simulink model "Cp_Lambda_Calculation"  (R2025a)
settings: Solver=FixedStepDiscrete  StartTime=0.0  StopTime=0  RelTol=1e-3
settings Model: Creator=Venkatesh  LastModifiedBy=lcrsb
settings SolverCC: AlgebraicLoopSolver=TrustRegion
settings DataIOCC: LimitDataPoints=on  SaveFormat=Array  ReturnWorkspaceOutputs=off
settings OptimizationCC: DefaultParameterBehavior=Inlined  UseDivisionForNetSlopeComputation=on  GainParamInheritBuiltInType=on  UseFloatMulNetSlope=on  InlineInvariantSignals=on  PassReuseOutputArgsAs=Individual arguments  ZeroExternalMemoryAtStartup=off  ZeroInternalMemoryAtStartup=off  NoFixptDivByZeroProtection=on  EfficientFloat2IntCast=on  LifeSpan=1  OptimizeBlockOrder=speed  DifferentSizesBufferReuse=on  EfficientTunableParamExpr=on
settings DebuggingCC: ParameterTunabilityLossMsg=error  UnconnectedInputMsg=warning  UnconnectedOutputMsg=warning  UnconnectedLineMsg=warning  SFUnexpectedBacktrackingDiag=warning  SFNoUnconditionalDefaultTransitionDiag=warning  SFExecutionAtInitializationDiag=none  ArithmeticOperatorsInVariantConditions=warning
settings HardwareCC: ProdLongLongMode=on
settings ModelReferenceCC: PropagateSignalLabelsOutOfModel=off
settings SFSimCC: SimUseLocalCustomCode=off  MATLABDynamicMemAlloc=off  CustomCodeUndefinedFunction=UseInterfaceOnly
settings RTWCC: SystemTargetFile=ert.tlc  TemplateMakefile=ert_default_tmf  RTWUseLocalCustomCode=off  GPUComputeCapability=3.5  Description=Embedded Coder
settings CodeAppCC: ForceParamTrailComments=on  IgnoreCustomStorageClasses=off  OperatorAnnotations=on  SimulinkDataObjDesc=on  SFDataObjDesc=on  CustomSymbolStrGlobalVar=rt$N$M  CustomSymbolStrType=$N$M  CustomSymbolStrFcn=$N$M$F  CustomSymbolStrMacro=$N$M  InsertBlockDesc=on
settings ERTTargetCC: ExtModeTransport=0.0  ExtModeStaticAlloc=off  ExtModeMexFile=ext_comm  ExtModeIntrfLevel=Level1  ERTCustomFileTemplate=example_file_process.tlc  ERTFilePackagingFormat=CompactWithDataFile  GenerateSampleERTMain=on  IncludeMdlTerminateFcn=off  CombineSignalStateStructs=on  SuppressErrorStatus=on  SupportAbsoluteTime=off  SupportComplex=off
settings ConfigComp: CovMetricSettings=dw  CovSaveCumulativeToWorkspaceVar=on  CovSaveSingleToWorkspaceVar=on  CovExternalEMLEnable=off  CovSFcnEnable=off

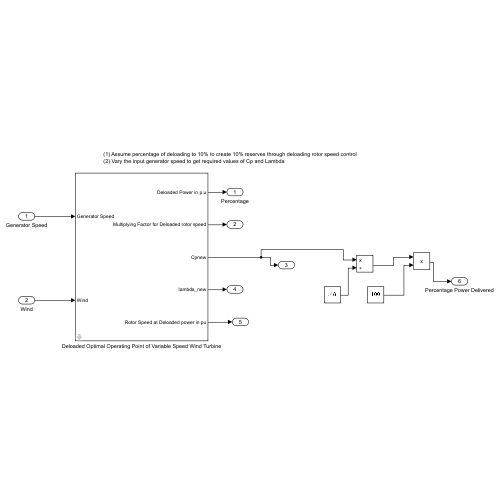
[thumbnail: Simulink's stored preview of the top-level diagram]
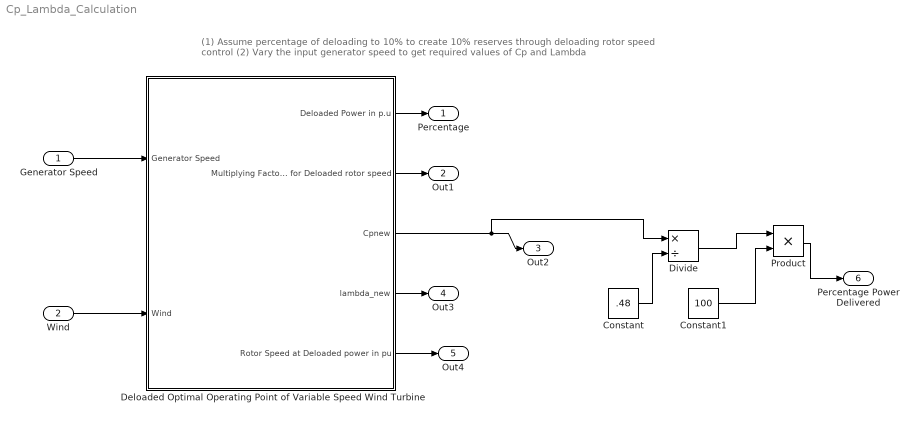
== system Cp_Lambda_Calculation ==
  note: (1) Assume percentage of deloading to 10% to create 10% reserves through deloading rotor speed control
      | (2) Vary the input generator speed to get required values of Cp and Lambda
  Generator Speed : Inport
  Wind : Inport  Port=2
  Constant : Constant  Value=.48
  Constant1 : Constant  Value=100
  Deloaded Optimal Operating Point of Variable Speed Wind Turbine : Subsystem  mask(Deloaded Optimal Operating Point Calculation){per_del=10, Generator_Speed=1.4207, Wind_Speed=12, Speed_MPPT=1.2, cp_opt=.4781, lambda_opt=8.3869, wind_base=12, speed_nom=1.2, lambda_nom=8.1, cp_nom=.48, beta=0}
      mask prompts: per_del "Percentage of Deloading"; Generator_Speed "Measured/Input Generator Speed p.u."; Wind_Speed "Wind Speed in m/s"; Speed_MPPT "Rotor Speed at MPPT in pu"; cp_opt "Optimum Power Coefficient"; lambda_opt "Optimum Tip Speed Ratio"; wind_base "Base Wind Speed in m/s"; speed_nom "Nominal Generator Speed p.u."; lambda_nom "Nominal Tip Speed Ratio"; cp_nom "Nominal Power Coefficient"; beta "Pitch Angle in degrees"
      mask help:
      | This block calculates the inputs required for the equation# 23 taken from the following reference:
      | []R.G. de Almeida, E. D. Castronuovo, and J. A. Peyas Lopes, “Optimum generation control in wind parks when carrying out system operator requests,” IEEE Trans. Power Syst., vol. 21, no. 2, pp. 718-725, May. 2006
  Divide : Product  Inputs=*/
  Product : Product
  Percentage : Outport
  Out1 : Outport  Port=2
  Out2 : Outport  Port=3
  Out3 : Outport  Port=4
  Out4 : Outport  Port=5
  Percentage Power Delivered : Outport  Port=6
  wires:
  Deloaded Optimal Operating Point of Variable Speed Wind Turbine/1(Deloaded Power in p.u) -> Percentage/1
  Deloaded Optimal Operating Point of Variable Speed Wind Turbine/2(Multiplying Factor for Deloaded rotor speed) -> Out1/1
  Deloaded Optimal Operating Point of Variable Speed Wind Turbine/3(Cpnew) -> Out2/1, Divide/1
  Deloaded Optimal Operating Point of Variable Speed Wind Turbine/4(lambda_new) -> Out3/1
  Deloaded Optimal Operating Point of Variable Speed Wind Turbine/5(Rotor Speed at Deloaded power in pu) -> Out4/1
  Constant/1 -> Divide/2
  Product/1 -> Percentage Power Delivered/1
  Divide/1 -> Product/1
  Constant1/1 -> Product/2
  Generator Speed/1 -> Deloaded Optimal Operating Point of Variable Speed Wind Turbine/1(Generator Speed)
  Wind/1 -> Deloaded Optimal Operating Point of Variable Speed Wind Turbine/2(Wind)

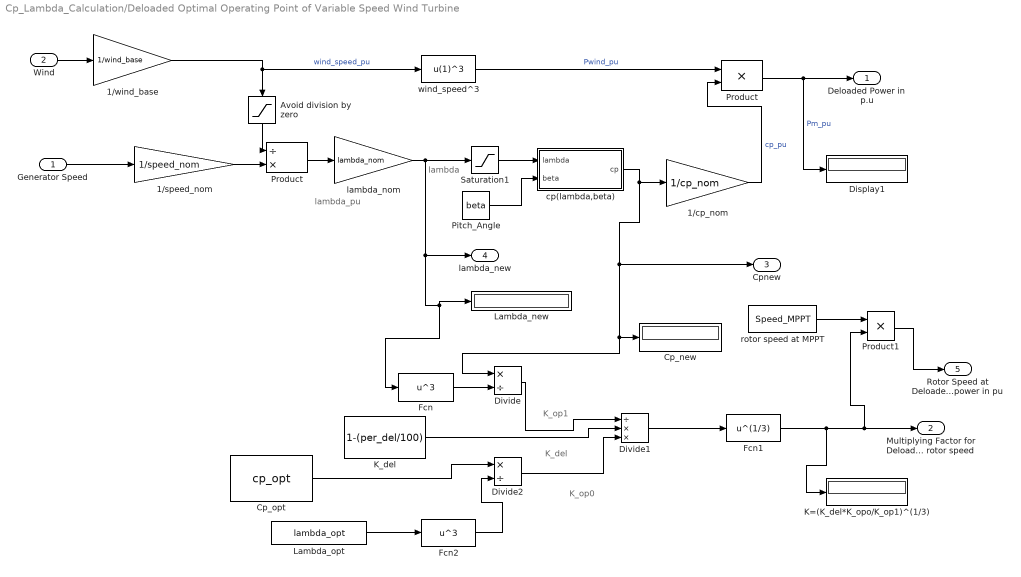
== system Cp_Lambda_Calculation/Deloaded Optimal Operating Point of Variable Speed Wind Turbine ==
  note: K_del
  note: K_op1
  note: K_op0
  note: lambda
  note: lambda_pu
  Generator Speed : Inport
  Wind : Inport  Port=2
  1/cp_nom : Gain  Gain=1/cp_nom  SaturateOnIntegerOverflow=on  OutDataTypeStr=Inherit: Same as input  ParamDataTypeStr=Inherit: Same as input
  "1/speed_nom " : Gain  Gain=1/speed_nom  SaturateOnIntegerOverflow=on  OutDataTypeStr=Inherit: Same as input  ParamDataTypeStr=Inherit: Same as input
  1/wind_base : Gain  Gain=1/wind_base  SaturateOnIntegerOverflow=on  OutDataTypeStr=Inherit: Same as input  ParamDataTypeStr=Inherit: Same as input
  "Avoid division by zero " : Saturate  UpperLimit=1e6  LowerLimit=1e-6
  Cp_new : Display
  Cp_opt : Constant  Value=cp_opt
  Display1 : Display
  Divide : Product  Inputs=*/
  Divide1 : Product  Inputs=/**
  Divide2 : Product  Inputs=*/
  Fcn : Fcn  Expr=u^3
  Fcn1 : Fcn  Expr=u^(1/3)
  Fcn2 : Fcn  Expr=u^3
  K=(K_del*K_opo/K_op1)^(1/3) : Display
  K_del : Constant  Value=1-(per_del/100)
  Lambda_new : Display
  Lambda_opt : Constant  Value=lambda_opt
  Pitch_Angle : Constant  Value=beta
  Product : Product  Inputs=/*  SaturateOnIntegerOverflow=on  OutDataTypeStr=Inherit: Same as first input
  "Product " : Product  SaturateOnIntegerOverflow=on  OutDataTypeStr=Inherit: Same as first input
  Product1 : Product
  Saturation1 : Saturate  UpperLimit=inf  LowerLimit=1e-6
  cp(lambda,beta) : Subsystem
  lambda_nom : Gain  Gain=lambda_nom  SaturateOnIntegerOverflow=on  OutDataTypeStr=Inherit: Same as input  ParamDataTypeStr=Inherit: Same as input
  rotor speed at MPPT : Constant  Value=Speed_MPPT
  wind_speed^3 : Fcn  Expr=u(1)^3
  Deloaded Power in p.u : Outport
  Multiplying Factor for Deloaded rotor speed : Outport  Port=2
  Cpnew : Outport  Port=3
  lambda_new : Outport  Port=4
  Rotor Speed at Deloaded power in pu : Outport  Port=5
  wires:
  Pitch_Angle/1 -> cp(lambda,beta)/2(beta)
  cp(lambda,beta)/1(cp) -> Cpnew/1, Divide/1, Cp_new/1, 1/cp_nom/1
  wind_speed^3/1 -> "Product "/1  "Pwind_pu"
  Wind/1 -> 1/wind_base/1
  Generator Speed/1 -> "1/speed_nom "/1
  lambda_nom/1 -> Saturation1/1, lambda_new/1, Fcn/1, Lambda_new/1
  1/cp_nom/1 -> "Product "/2  "cp_pu"
  Saturation1/1 -> cp(lambda,beta)/1(lambda)
  Product/1 -> lambda_nom/1
  1/wind_base/1 -> wind_speed^3/1, "Avoid division by zero "/1  "wind_speed_pu"
  "Avoid division by zero "/1 -> Product/1
  "1/speed_nom "/1 -> Product/2
  "Product "/1 -> Display1/1, Deloaded Power in p.u/1  "Pm_pu"
  Fcn/1 -> Divide/2
  Divide/1 -> Divide1/1
  Divide1/1 -> Fcn1/1
  K_del/1 -> Divide1/2
  Cp_opt/1 -> Divide2/1
  Divide2/1 -> Divide1/3
  Lambda_opt/1 -> Fcn2/1
  Fcn1/1 -> Product1/2, Multiplying Factor for Deloaded rotor speed/1, K=(K_del*K_opo/K_op1)^(1/3)/1
  Fcn2/1 -> Divide2/2
  Product1/1 -> Rotor Speed at Deloaded power in pu/1
  rotor speed at MPPT/1 -> Product1/1

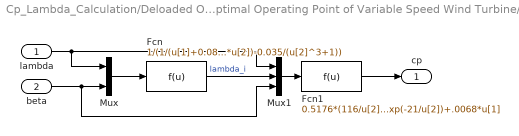
== system Cp_Lambda_Calculation/Deloaded Optimal Operating Point of Variable Speed Wind Turbine/cp(lambda,beta) ==
  lambda : Inport
  beta : Inport  Port=2
  Fcn : Fcn  Expr=1/(1/(u[1]+0.08*u[2])-0.035/(u[2]^3+1))
  Fcn1 : Fcn  Expr=0.5176*(116/u[2]-.4*u[3]-5)*exp(-21/u[2])+.0068*u[1]
  Mux : Mux  Inputs=2
  Mux1 : Mux  Inputs=3
  cp : Outport
  wires:
  Fcn/1 -> Mux1/2  "lambda_i"
  Fcn1/1 -> cp/1
  lambda/1 -> Mux1/1, Mux/1
  Mux1/1 -> Fcn1/1
  beta/1 -> Mux1/3, Mux/2
  Mux/1 -> Fcn/1
